simulink model "first"  (R2019b)
settings: Solver=VariableStepAuto  StartTime=0.0  StopTime=20  RelTol=1e-3
undefined symbols (not defined in the file or in its folder): Earth, WGS84
libraries: dspsrcs4 x3, aerolibfltsims x2, aerolibtransform2 x1
settings Model: Creator=LENOVO  LastModifiedBy=LENOVO
settings DataIOCC: ExternalInput=[time, x_konum, z_konum]
settings OptimizationCC: BlockReduction=off  DefaultParameterBehavior=Inlined  BufferReuse=off

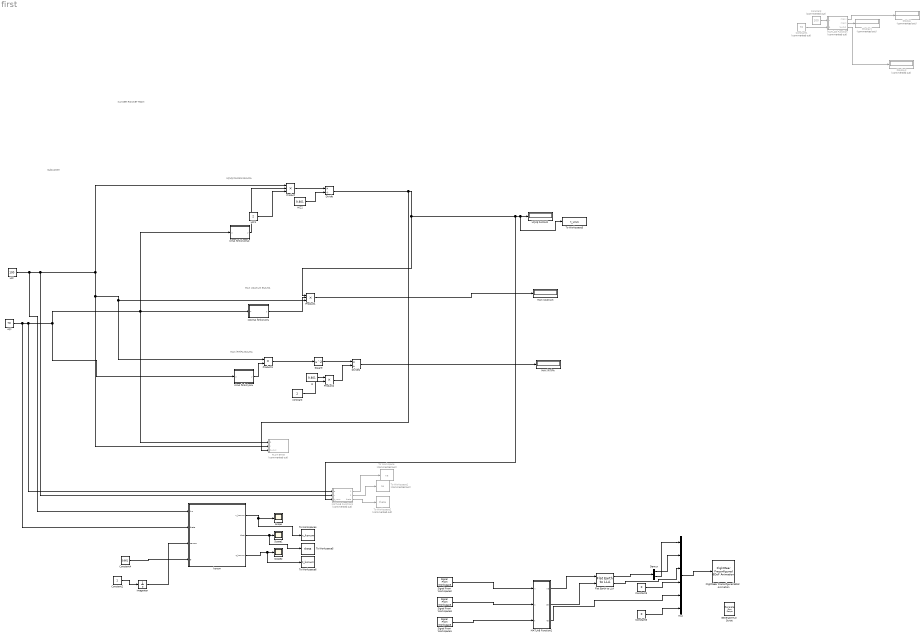
== system first ==
  note: Subsystem
  note: KAYZER ROCKET TEAM
  note: UÇUŞ ZAMANI BULMA
  note: MAX UZAKLIK BULMA
  note: MAX İRTİFA BULMA
  AÇI : Constant  Value=70
  Constant : Constant  Commented=on  Value=100
  Constant1 : Constant  Commented=on  Value=70
  Constant2 : Constant
  Constant3 : Constant  Value=0
  Constant4 : Constant  Value=9.801
  Constant5 : Constant  Value=0
  Demux : Demux  Outputs=2
  Display : Display  Commented=on
  Display1 : Display  Commented=on
  Display2 : Display  Commented=on
  Divide : Product  Inputs=*/
  Divide1 : Product  Inputs=*/
  Flat Earth to LLA : aerolibtransform2/Flat Earth to LLA  units=Metric (MKS)  ptype=Earth (WGS84)  F=1/298.257223563  R=6378137  LL0=[0 10]  psi=0
  FlightGear Preconfigured 6DoF Animation : aerolibfltsims/FlightGear Preconfigured 6DoF Animation  xFlightGearVersion=v2018.3  DestinationIpAddress=127.0.0.1  DestinationPort=5502  SampleTime=1/30  packetVersion=24
      settings: SourceProductName=Aerospace Blockset
  Generate Run Script : aerolibfltsims/Generate Run Script  Architecture=Win64  dataFlow=Send  GeometryModelName=milal  AirportId=KSFO  RunwayId=10L  InitialAltitude=7224  InitialHeading=113  OffsetDistance=4.72  OffsetAzimuth=0  InstallScenery=on  DisableShaders=off  OriginAddress=127.0.0.1  DestinationPort=5502  OriginPort=5505  LocalAddress=127.0.0.1  OutputFileName=runfg.bat  FlightGearBaseDirectory=C:\Program Files\FlightGear 2020.3
  HIZ : Constant  Value=100
  HIZ1 : Constant  Value=2
  HIZ2 : Constant  Value=9.801
  Integrator : Integrator  LimitOutput=on  UpperSaturationLimit=19.18
  MATLAB Function : MATLAB Function  Commented=on  TreatAsAtomicUnit=on
  MATLAB Function1 : MATLAB Function  Commented=on  TreatAsAtomicUnit=on
  MATLAB Function2 : MATLAB Function  TreatAsAtomicUnit=on
  MAX UZAKLIK : Display
  MAX İRTİFA : Display
  Mux : Mux  Inputs=6
  PLOT ETME : MATLAB Function  Commented=on  TreatAsAtomicUnit=on
  Product : Product  Inputs=3
  Product1 : Product  Inputs=3
  Product2 : Product
  Product3 : Product
  Scope : Scope
  Scope1 : Scope
  Scope2 : Scope
  Signal From Workspace1 : dspsrcs4/Signal From Workspace  X=out.theta  Ts=0.1  nsamps=1  OutputAfterFinalValue=Setting to zero  ignoreOrWarnInputAndFrameLengths=off  OutputFrames=off
  Signal From Workspace2 : dspsrcs4/Signal From Workspace  X=out.x_konum  Ts=0.1  nsamps=1  OutputAfterFinalValue=Setting to zero  ignoreOrWarnInputAndFrameLengths=off  OutputFrames=off
  Signal From Workspace3 : dspsrcs4/Signal From Workspace  X=out.z_konum  Ts=0.1  nsamps=1  OutputAfterFinalValue=Setting to zero  ignoreOrWarnInputAndFrameLengths=off  OutputFrames=off
  Square : Math  Operator=square  SignedPower=off  SaturateOnIntegerOverflow=on
  To Workspace : ToWorkspace  Commented=on  VariableName=xe  SampleTime=0.1
      settings: Save2DSignal=2-D array (concatenate along first dimension)
  To Workspace1 : ToWorkspace  Commented=on  VariableName=ze  SampleTime=0.1
      settings: Save2DSignal=2-D array (concatenate along first dimension)
  To Workspace2 : ToWorkspace  Commented=on  VariableName=theta  SampleTime=0.1
      settings: Save2DSignal=2-D array (concatenate along first dimension)
  To Workspace3 : ToWorkspace  VariableName=t_ucus  SaveFormat=Timeseries  SampleTime=-1
  To Workspace4 : ToWorkspace  VariableName=x_konum  SampleTime=0.1
      settings: Save2DSignal=2-D array (concatenate along first dimension)
  To Workspace5 : ToWorkspace  VariableName=theta  SampleTime=0.1
      settings: Save2DSignal=2-D array (concatenate along first dimension)
  To Workspace6 : ToWorkspace  VariableName=z_konum  SampleTime=0.1
      settings: Save2DSignal=2-D array (concatenate along first dimension)
  UÇUŞ ZAMANI : Display
  "constant " : Constant  Value=2
  cosinus fonksiyonu : MATLAB Function  TreatAsAtomicUnit=on
  g : Constant  Value=9.801
  konum : Subsystem
  sinus fonksiyonu : MATLAB Function  TreatAsAtomicUnit=on
  sinus fonksiyonu2 : MATLAB Function  TreatAsAtomicUnit=on
  wires:
  Constant1/1 -> MATLAB Function/2(a)
  Constant/1 -> MATLAB Function/1(v)
  MATLAB Function/1(maxx) -> Display/1
  MATLAB Function/3(t_ucus) -> Display2/1
  MATLAB Function/2(maxz) -> Display1/1
  Divide/1 -> Product1/1, MATLAB Function1/3(t_ucus), To Workspace3/1, UÇUŞ ZAMANI/1, PLOT ETME/3(t_ucus)
  Product1/1 -> MAX UZAKLIK/1
  Divide1/1 -> MAX İRTİFA/1
  sinus fonksiyonu/1(y) -> Product3/2
  Product2/1 -> Divide1/2
  Product3/1 -> Square/1
  "constant "/1 -> Product2/2
  Square/1 -> Divide1/1
  g/1 -> Product2/1
  cosinus fonksiyonu/1(y) -> Product1/2
  HIZ1/1 -> Product/3
  Product/1 -> Divide/1
  sinus fonksiyonu2/1(y) -> Product/2
  AÇI/1 -> konum/2(theta), MATLAB Function1/1(a), PLOT ETME/1(a), cosinus fonksiyonu/1(u), sinus fonksiyonu2/1(u), sinus fonksiyonu/1(u)
  HIZ/1 -> konum/1(hız), MATLAB Function1/2(v), Product/1, PLOT ETME/2(v), Product3/1, Product1/3
  HIZ2/1 -> Divide/2
  Flat Earth to LLA/1 -> Demux/1
  Mux/1 -> FlightGear Preconfigured 6DoF Animation/1
  Demux/1 -> Mux/2
  Demux/2 -> Mux/1
  Flat Earth to LLA/2 -> Mux/3
  Constant3/1 -> Mux/4
  MATLAB Function2/2(ze) -> Flat Earth to LLA/2
  Signal From Workspace3/1 -> MATLAB Function2/2(z)
  Signal From Workspace2/1 -> MATLAB Function2/1(x)
  MATLAB Function2/1(xe) -> Flat Earth to LLA/1
  MATLAB Function2/3(te) -> Mux/5
  Constant5/1 -> Mux/6
  MATLAB Function1/1(x_konum) -> To Workspace/1
  MATLAB Function1/3(theta) -> To Workspace2/1
  MATLAB Function1/2(z_konum) -> To Workspace1/1
  Signal From Workspace1/1 -> MATLAB Function2/3(t)
  Constant2/1 -> Integrator/1
  Integrator/1 -> konum/3(zaman)
  Constant4/1 -> konum/4(g)
  konum/3(z_konum) -> To Workspace6/1, Scope2/1
  konum/2(thet) -> To Workspace5/1, Scope1/1
  konum/1(x_konum) -> To Workspace4/1, Scope/1

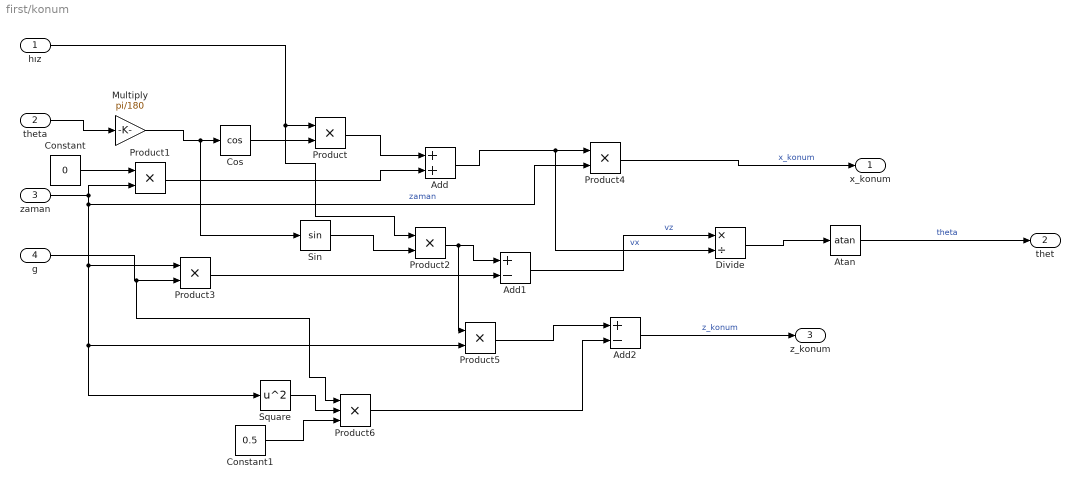
== system first/konum ==
  hız : Inport
  theta : Inport  Port=2
  zaman : Inport  Port=3
  g : Inport  Port=4
  Add : Sum
  Add1 : Sum  Inputs=+-
  Add2 : Sum  Inputs=+-
  Atan : Trigonometry  Operator=atan
  Constant : Constant  Value=0
  Constant1 : Constant  Value=0.5
  Cos : Trigonometry  Operator=cos
  Divide : Product  Inputs=*/
  Multiply : Gain  Gain=pi/180
  Product{,1..5} (6 alike) : Product
  Product6 : Product  Inputs=3
  Sin : Trigonometry
  Square : Math  Operator=square  SignedPower=off  SaturateOnIntegerOverflow=on
  x_konum : Outport
  thet : Outport  Port=2
  z_konum : Outport  Port=3
  wires:
  theta/1 -> Multiply/1
  Multiply/1 -> Sin/1, Cos/1
  hız/1 -> Product2/1, Product/1
  Cos/1 -> Product/2
  zaman/1 -> Product4/2, Square/1, Product5/2, Product3/1, Product1/2  "zaman"
  Constant/1 -> Product1/1
  Product1/1 -> Add/2
  Product/1 -> Add/1
  Add/1 -> Divide/2, Product4/1  "vx"
  Sin/1 -> Product2/2
  g/1 -> Product6/1, Product3/2
  Product3/1 -> Add1/2
  Product2/1 -> Product5/1, Add1/1
  Add1/1 -> Divide/1  "vz"
  Product4/1 -> x_konum/1  "x_konum"
  Product5/1 -> Add2/1
  Constant1/1 -> Product6/3
  Square/1 -> Product6/2
  Product6/1 -> Add2/2
  Add2/1 -> z_konum/1  "z_konum"
  Divide/1 -> Atan/1
  Atan/1 -> thet/1  "theta"

== matlab function first/PLOT ETME ==
  data: a input; v input; t_ucus input
function fcn(a,v,t_ucus)
for t=0:0.1:t_ucus
time=0:0.01:t;
g=9.801; %yerçekimi ivmesi
vx=v*cosd(a);
x_konum=vx.*time;
z_konum=(v*sind(a).*time) - (1/2).*g.*(time.^2);
[maxx,idx] = max(x_konum);
[maxz,idz] = max(z_konum);
plot(x_konum,z_konum,x_konum(idx),z_konum(idx),'pr');
%   set('xLim',[0 1000]);
%   set('yLim',[0 600]);
% legend(sprintf('Max İrtifa = %0.3f',maxz),sprintf('Maximum Uzaklık = %0.3f',maxx));
% axis([xlim min(x_konum) max(x_konum)+1]);
trxt=('Max Uzaklık');
txt=('Maximum İrtifa \uparrow');
 text(x_konum(idx),z_konum(idx),trxt,'VerticalAlignment','bottom');
 text(x_konum(idz),maxz,txt,'HorizontalAlignment','right');
 if t==t_ucus
     break
 end
drawnow;
end

end

== matlab function first/MATLAB Function ==
  data: v input; maxx output; a input; maxz output; t_ucus output
function [maxx,maxz,t_ucus] = fcn(v,a)
g=9.801; %yerçekimi ivmesi
t_ucus=(2*v*sind(a))/g;
t_cikis=t_ucus/2;
time=0:0.01:t_ucus;
vx=v*cosd(a);
vz=v*sind(a)-g*time;
max_irtifa=(v*sind(a)^2)/(2*g);
max_uzaklik=v*cosd(a).*t_ucus;
x_konum=vx.*time;
z_konum=(v*sind(a).*time) - (1/2).*g.*(time.^2);
% plot(x_konum,z_konum);

[maxx,idx] = max(x_konum);
[maxz,idz] = max(z_konum);
plot(x_konum,z_konum,x_konum(idx),z_konum(idx),'pr');
% legend(sprintf('Max İrtifa = %0.3f',maxz),sprintf('Maximum Uzaklık = %0.3f',maxx));
% axis([xlim min(x_konum) max(x_konum)+1]);
% trxt=('Max Uzaklık');
% txt=('Maximum İrtifa \uparrow');
%  text(x_konum(length(time)),z_konum(length(time)),trxt,'VerticalAlignment','bottom');
%  text(x_konum(idz),maxz,txt,'HorizontalAlignment','right');
end

== matlab function first/sinus fonksiyonu2 ==
  data: u input; y output
function y = fcn(u)

y = sind(u);
end

== matlab function first/cosinus fonksiyonu ==
  data: u input; y output
function y = fcn(u)

y = cosd(u);
end

== matlab function first/sinus fonksiyonu ==
  data: u input; y output
function y = fcn(u)

y = sind(u);
end

== matlab function first/MATLAB Function1 ==
  data: a input; v input; t_ucus input; x_konum output double; z_konum output double; theta output double
function [x_konum,z_konum,theta]=fcn(a,v,t_ucus)
time=0:0.1:round(t_ucus);
g=9.801; %yerçekimi ivmesi
vx=v*cosd(a)+0.*time;
x_konum=vx.*time;
z_konum=(v*sind(a).*time) - (1/2).*g.*(time.^2);
vz=v*sind(a)-g.*time;
theta=atan(vz./vx);
end

== matlab function first/MATLAB Function2 ==
  data: x input; xe output; z input; ze output; t input; te output
function [xe,ze,te] = fcn(x,z,t)
xe=-4*[x(1,1) ;0 ; 0];
ze=-2*(z(1,1)+15);
te=-t(1,1)+pi/2;
end
